simulink model "controls_testing"  (R2025b)
settings: Solver=VariableStepAuto  StartTime=0.0  StopTime=10  RelTol=1e-3
libraries: simulink x2, controls x1
settings Model: Creator=jessi  LastModifiedBy=fabiy

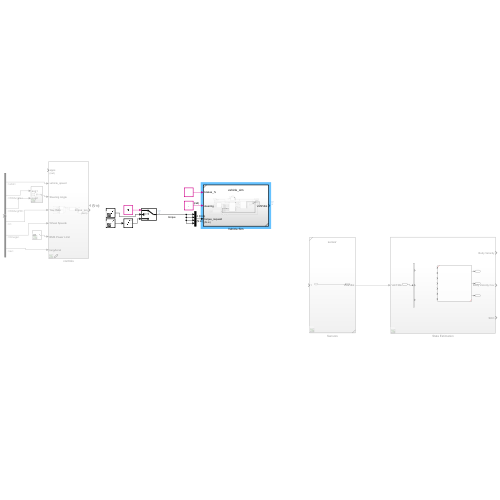
[thumbnail: Simulink's stored preview of the top-level diagram]
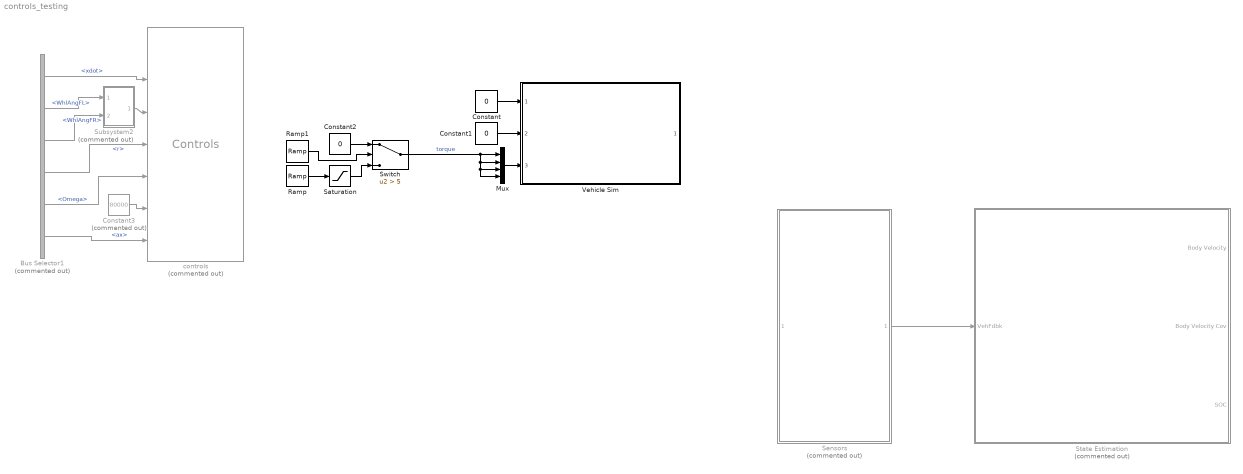
== system controls_testing ==
  Bus Selector1 : BusSelector  Commented=on  OutputSignals=BdyFrm.Cg.Vel.xdot,BdyFrm.FrntAxl.Steer.WhlAngFL,BdyFrm.FrntAxl.Steer.WhlAngFR,BdyFrm.Cg.AngVel.r,Wheels.Omega,BdyFrm.Cg.Acc.ax
  Constant : Constant  Value=0
  Constant1 : Constant  Value=0
  Constant2 : Constant  Value=0
  Constant3 : Constant  Commented=on  Value=80000
  Mux : Mux
  Ramp : simulink/Sources/Ramp  slope=10/(0.7)  start=0  InitialOutput=0
  Ramp1 : simulink/Sources/Ramp  slope=1  start=0  InitialOutput=0
  Saturation : Saturate  UpperLimit=10  LowerLimit=0
  Sensors : Subsystem  Commented=on  ReferencedSubsystem=sensor
  State Estimation : Subsystem  Commented=on
  Subsystem2 : Subsystem  Commented=on
  Switch : Switch  Criteria=u2 > Threshold  Threshold=5  SaturateOnIntegerOverflow=off  InputSameDT=off
  Vehicle Sim : Subsystem  ReferencedSubsystem=vehicle_sim
  controls : controls/Controls  Commented=on  SystemSampleTime=-1  VariantActivationTime=update diagram  EmptyChoice=off  PassThrough=off  PassThroughVariantControl=(default)  EmptyChoiceVariantControl=(default)  AllowFlexibleInterface=on  Latency=0  AutoFrameSizeCalculation=off
  wires:
  Constant/1 -> Vehicle Sim/1
  Constant1/1 -> Vehicle Sim/2
  Bus Selector1/3 -> Subsystem2/2(ang2)  "<WhlAngFR>"
  Bus Selector1/1 -> controls/2  "<xdot>"
  Constant3/1 -> controls/6
  Bus Selector1/2 -> Subsystem2/1(ang1)  "<WhlAngFL>"
  Bus Selector1/5 -> controls/5  "<Omega>"
  Subsystem2/1(Out1) -> controls/3
  Bus Selector1/4 -> controls/4  "<r>"
  Bus Selector1/6 -> controls/7  "<ax>"
  Sensors/1 -> State Estimation/1(VehFdbk)
  Saturation/1 -> Switch/3
  Ramp/1 -> Saturation/1
  Mux/1 -> Vehicle Sim/3
  Switch/1 -> Mux/4, Mux/3, Mux/2, Mux/1  "torque"
  Ramp1/1 -> Switch/2
  Constant2/1 -> Switch/1

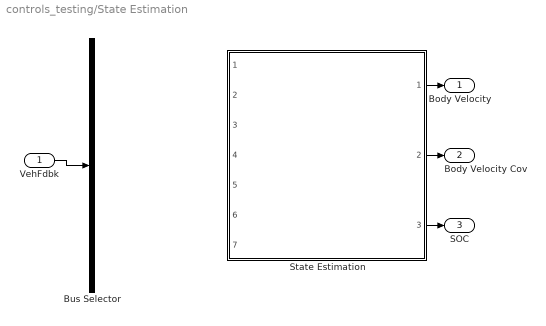
== system controls_testing/State Estimation ==
  VehFdbk : Inport
  Bus Selector : BusSelector  OutputSignals=BdyFrm.Cg.Acc.ax,BdyFrm.Cg.Acc.ay,BdyFrm.Cg.AngVel.r
  State Estimation : Subsystem  ReferencedSubsystem=state_estimation
  Body Velocity : Outport
  Body Velocity Cov : Outport  Port=2
  SOC : Outport  Port=3
  wires:
  State Estimation/3 -> SOC/1
  State Estimation/2 -> Body Velocity Cov/1
  State Estimation/1 -> Body Velocity/1
  VehFdbk/1 -> Bus Selector/1

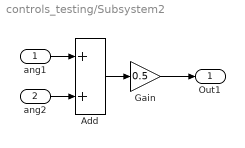
== system controls_testing/Subsystem2 ==
  ang1 : Inport
  ang2 : Inport  Port=2
  Add : Sum
  Gain : Gain  Gain=0.5
  Out1 : Outport
  wires:
  ang2/1 -> Add/2
  ang1/1 -> Add/1
  Add/1 -> Gain/1
  Gain/1 -> Out1/1
